simulink model "drone_PID"  (R2023a)
settings: Solver=ode4  StartTime=0.0  StopTime=10  FixedStep=0.01  RelTol=1e-3
values from neighbouring files (symbols this model uses):
  g = 9.807    [dxdt.m]    (also in main.m)
  m = 2.5    [dxdt.m]    (also in main.m)
  x0 = [0, 5, 0, 0, 0, 0]    [main.m]
undefined symbols (not defined in the file or in its folder): dxdt, Kp_omega, Kp_theta, Kp_vx, Kp_vy, Kp_x, Kp_y
settings Model: Creator=timme  LastModifiedBy=timme
settings OptimizationCC: BlockReduction=off  DefaultParameterBehavior=Inlined  BufferReuse=off

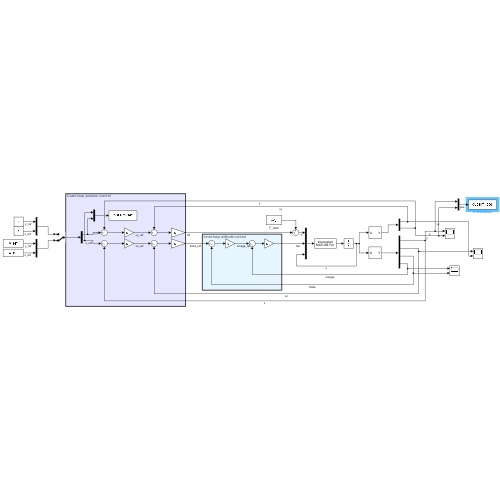
[thumbnail: Simulink's stored preview of the top-level diagram]
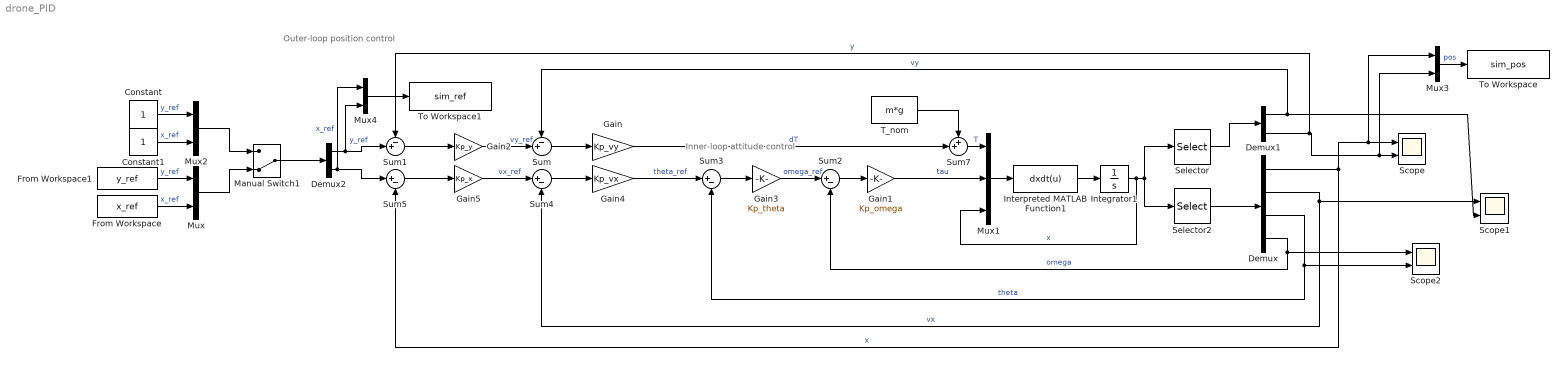
== system drone_PID ==
  note: Outer-loop position control
  note: Inner-loop attitude control
  Constant : Constant
  Constant1 : Constant
  Demux : Demux
  Demux1 : Demux  Outputs=2
  Demux2 : Demux  Outputs=2
  From Workspace : FromWorkspace  VariableName=x_ref
  From Workspace1 : FromWorkspace  VariableName=y_ref
  Gain : Gain  Gain=Kp_vy
  Gain1 : Gain  Gain=Kp_omega
  Gain2 : Gain  Gain=Kp_y
  Gain3 : Gain  Gain=Kp_theta
  Gain4 : Gain  Gain=Kp_vx
  Gain5 : Gain  Gain=Kp_x
  Integrator1 : Integrator  InitialCondition=x0
  Interpreted MATLAB Function1 : MATLABFcn  MATLABFcn=dxdt(u)  OutputDimensions=6
  Manual Switch1 : ManualSwitch  CurrentSetting=0
  Mux{,2..4} (4 alike) : Mux  Inputs=2
  Mux1 : Mux  Inputs=3
  Scope : Scope  NumInputPorts=2
  Scope1 : Scope  NumInputPorts=2
  Scope2 : Scope  NumInputPorts=2
  Selector : Selector  InputPortWidth=6  IndexOptions=Index vector (dialog)  Indices=[5 2]  OutputSizes=1
  Selector2 : Selector  InputPortWidth=6  IndexOptions=Index vector (dialog)  Indices=[1 4 3 6]  OutputSizes=1
  Sum : Sum  Inputs=-+|
  Sum1 : Sum  Inputs=-+|
  Sum{2..5} (4 alike) : Sum  Inputs=|+-
  Sum7 : Sum  Inputs=++|
  T_nom : Constant  Value=m*g
  To Workspace : ToWorkspace  VariableName=sim_pos  SaveFormat=Timeseries  SampleTime=0.01
      settings: Decimation=2
  To Workspace1 : ToWorkspace  VariableName=sim_ref  SaveFormat=Timeseries  SampleTime=-1
  wires:
  Interpreted MATLAB Function1/1 -> Integrator1/1
  Sum4/1 -> Gain4/1
  Demux/1 -> Sum5/2, Mux3/1, Scope/1  "x"
  Mux1/1 -> Interpreted MATLAB Function1/1
  Integrator1/1 -> Selector2/1, Selector/1, Mux1/3  "x"
  Gain5/1 -> Sum4/1  "vx_ref"
  Demux1/1 -> Sum/1, Scope1/2  "vy"
  Sum2/1 -> Gain1/1
  Gain1/1 -> Mux1/2  "tau"
  Sum/1 -> Gain/1
  Selector/1 -> Demux1/1
  Sum3/1 -> Gain3/1
  From Workspace/1 -> Mux/2  "x_ref"
  Selector2/1 -> Demux/1
  Sum5/1 -> Gain5/1
  Sum1/1 -> Gain2/1
  Gain4/1 -> Sum3/1  "theta_ref"
  Demux2/1 -> Mux4/2, Sum1/2  "y_ref"
  Demux/3 -> Sum3/2, Scope2/2  "theta"
  Gain/1 -> Sum7/2  "dT"
  T_nom/1 -> Sum7/1
  Demux/4 -> Sum2/2, Scope2/1  "omega"
  Gain2/1 -> Sum/2  "vy_ref"
  Demux1/2 -> Mux3/2, Scope/2, Sum1/1  "y"
  Gain3/1 -> Sum2/1  "omega_ref"
  Sum7/1 -> Mux1/1  "T"
  Demux/2 -> Sum4/2, Scope1/1  "vx"
  From Workspace1/1 -> Mux/1  "y_ref"
  Constant1/1 -> Mux2/2  "x_ref"
  Constant/1 -> Mux2/1  "y_ref"
  Demux2/2 -> Sum5/1, Mux4/1  "x_ref"
  Manual Switch1/1 -> Demux2/1
  Mux/1 -> Manual Switch1/2
  Mux2/1 -> Manual Switch1/1
  Mux3/1 -> To Workspace/1  "pos"
  Mux4/1 -> To Workspace1/1
